simulink model "case1"  (R2024b)
settings: Solver=FixedStepAuto  StartTime=0  StopTime=1  FixedStep=1e-7  RelTol=1e-3
values from neighbouring files (symbols this model uses):
  SG_D_1_D = 0.01056    [IEEE9_case_parameters.m]    (also in case1_parameters.m; case2_parameters.m; case3_parameters.m; case4_parameters.m)
  SG_D_1_EnableSaturation = 0    [IEEE9_case_parameters.m]    (also in case1_parameters.m; case2_parameters.m; case3_parameters.m; case4_parameters.m)
  SG_D_1_f0 = 60    [IEEE9_case_parameters.m]    (also in case1_parameters.m; case2_parameters.m; case3_parameters.m; case4_parameters.m)
  SG_D_1_H = 7.5    [IEEE9_case_parameters.m]    (also in case1_parameters.m; case2_parameters.m; case3_parameters.m; case4_parameters.m)
  SG_D_1_K_A = 20    [IEEE9_case_parameters.m]    (also in case1_parameters.m; case2_parameters.m; case3_parameters.m; case4_parameters.m)
  SG_D_1_K_E = 1.000000e+1    (= 10)    [IEEE9_case_parameters.m]    (also in case1_parameters.m; case2_parameters.m; case3_parameters.m; case4_parameters.m)
  SG_D_1_K_F = 2.363    [IEEE9_case_parameters.m]    (also in case1_parameters.m; case2_parameters.m; case3_parameters.m; case4_parameters.m)
  SG_D_1_K_s = 0.5    [IEEE9_case_parameters.m]    (also in case1_parameters.m = 5; case2_parameters.m = 5; case3_parameters.m = 5; case4_parameters.m = 5)
  SG_D_1_R_a = 0.001088    [IEEE9_case_parameters.m]    (also in case1_parameters.m; case2_parameters.m; case3_parameters.m; case4_parameters.m)
  SG_D_1_S_A = 1    [IEEE9_case_parameters.m]    (also in case1_parameters.m; case2_parameters.m; case3_parameters.m; case4_parameters.m)
  SG_D_1_S_B = 0.103    [IEEE9_case_parameters.m]    (also in case1_parameters.m; case2_parameters.m; case3_parameters.m; case4_parameters.m)
  SG_D_1_S_N = 10.659857    [IEEE9_case_parameters.m]    (also in case1_parameters.m; case2_parameters.m; case3_parameters.m; case4_parameters.m)
  SG_D_1_SpeedPara = 200    [IEEE9_case_parameters.m]    (also in case1_parameters.m; case2_parameters.m; case3_parameters.m; case4_parameters.m)
  SG_D_1_T_0 = 0.720173    [IEEE9_case_parameters.m]    (also in case1_parameters.m = 0.755522; case2_parameters.m = 0.808931; case3_parameters.m = 0.869402; case4_parameters.m = 0.729316)
  SG_D_1_T_1 = 0.3    [IEEE9_case_parameters.m]    (also in case1_parameters.m; case2_parameters.m; case3_parameters.m; case4_parameters.m)
  SG_D_1_T_2 = 0.05    [IEEE9_case_parameters.m]    (also in case1_parameters.m; case2_parameters.m; case3_parameters.m; case4_parameters.m)
  SG_D_1_T_3 = 0.02    [IEEE9_case_parameters.m]    (also in case1_parameters.m; case2_parameters.m; case3_parameters.m; case4_parameters.m)
  SG_D_1_T_4 = 0.005    [IEEE9_case_parameters.m]    (also in case1_parameters.m; case2_parameters.m; case3_parameters.m; case4_parameters.m)
  SG_D_1_T_A = 0.02    [IEEE9_case_parameters.m]    (also in case1_parameters.m; case2_parameters.m; case3_parameters.m; case4_parameters.m)
  SG_D_1_T_dd = 8.000000e+0    (= 8)    [IEEE9_case_parameters.m]    (also in case1_parameters.m; case2_parameters.m; case3_parameters.m; case4_parameters.m)
  SG_D_1_T_ddd = 0.04    [IEEE9_case_parameters.m]    (also in case1_parameters.m; case2_parameters.m; case3_parameters.m; case4_parameters.m)
  SG_D_1_T_E = 0.314    [IEEE9_case_parameters.m]    (also in case1_parameters.m; case2_parameters.m; case3_parameters.m; case4_parameters.m)
  SG_D_1_T_F = 0.35    [IEEE9_case_parameters.m]    (also in case1_parameters.m; case2_parameters.m; case3_parameters.m; case4_parameters.m)
  SG_D_1_T_qd = 0.8    [IEEE9_case_parameters.m]    (also in case1_parameters.m; case2_parameters.m; case3_parameters.m; case4_parameters.m)
  SG_D_1_T_qdd = 0.02    [IEEE9_case_parameters.m]    (also in case1_parameters.m; case2_parameters.m; case3_parameters.m; case4_parameters.m)
  SG_D_1_T_speed = 0.1    [IEEE9_case_parameters.m]    (also in case1_parameters.m = 200; case2_parameters.m = 200; case3_parameters.m = 200; case4_parameters.m = 200)
  SG_D_1_T_w = 0.5    [IEEE9_case_parameters.m]    (also in case1_parameters.m; case2_parameters.m; case3_parameters.m; case4_parameters.m)
  SG_D_1_V_ref = 1.990276    [IEEE9_case_parameters.m]    (also in case1_parameters.m = 2.042296; case2_parameters.m = 2.051388; case3_parameters.m = 2.089584; case4_parameters.m = 2.01845)
  SG_D_1_w_ref = 376.991118    [IEEE9_case_parameters.m]    (also in case1_parameters.m; case2_parameters.m; case3_parameters.m; case4_parameters.m)
  SG_D_1_wb = 6.000000e+1    (= 60)    [IEEE9_case_parameters.m]    (also in case1_parameters.m; case2_parameters.m; case3_parameters.m; case4_parameters.m)
  SG_D_1_x_d = 1.9    [IEEE9_case_parameters.m]    (also in case1_parameters.m; case2_parameters.m; case3_parameters.m; case4_parameters.m)
  SG_D_1_x_dd = 0.302    [IEEE9_case_parameters.m]    (also in case1_parameters.m; case2_parameters.m; case3_parameters.m; case4_parameters.m)
  SG_D_1_x_ddd = 0.204    [IEEE9_case_parameters.m]    (also in case1_parameters.m; case2_parameters.m; case3_parameters.m; case4_parameters.m)
  SG_D_1_x_l = 0.05    [IEEE9_case_parameters.m]    (also in case1_parameters.m; case2_parameters.m; case3_parameters.m; case4_parameters.m)
  SG_D_1_x_q = 1.3    [IEEE9_case_parameters.m]    (also in case1_parameters.m; case2_parameters.m; case3_parameters.m; case4_parameters.m)
  SG_D_1_x_qd = 0.5    [IEEE9_case_parameters.m]    (also in case1_parameters.m; case2_parameters.m; case3_parameters.m; case4_parameters.m)
  SG_D_1_x_qdd = 0.3    [IEEE9_case_parameters.m]    (also in case1_parameters.m; case2_parameters.m; case3_parameters.m; case4_parameters.m)
  SG_D_2_D = 0.02    [IEEE9_case_parameters.m]    (also in case1_parameters.m; case2_parameters.m; case3_parameters.m; case4_parameters.m)
  SG_D_2_EnableSaturation = 0    [IEEE9_case_parameters.m]    (also in case1_parameters.m; case2_parameters.m; case3_parameters.m; case4_parameters.m)
  SG_D_2_f0 = 60    [IEEE9_case_parameters.m]    (also in case1_parameters.m; case2_parameters.m; case3_parameters.m; case4_parameters.m)
  SG_D_2_H = 8.000000e+0    (= 8)    [IEEE9_case_parameters.m]    (also in case1_parameters.m; case2_parameters.m; case3_parameters.m; case4_parameters.m)
  SG_D_2_K_A = 20    [IEEE9_case_parameters.m]    (also in case1_parameters.m; case2_parameters.m; case3_parameters.m; case4_parameters.m)
  SG_D_2_K_E = 1.000000e+1    (= 10)    [IEEE9_case_parameters.m]    (also in case1_parameters.m; case2_parameters.m; case3_parameters.m; case4_parameters.m)
  SG_D_2_K_F = 2.363    [IEEE9_case_parameters.m]    (also in case1_parameters.m; case2_parameters.m; case3_parameters.m; case4_parameters.m)
  SG_D_2_K_s = 0.5    [IEEE9_case_parameters.m]    (also in case1_parameters.m = 4; case2_parameters.m = 4; case3_parameters.m = 4; case4_parameters.m = 4)
  SG_D_2_R_a = 0.001088    [IEEE9_case_parameters.m]    (also in case1_parameters.m; case2_parameters.m; case3_parameters.m; case4_parameters.m)
  SG_D_2_S_A = 1    [IEEE9_case_parameters.m]    (also in case1_parameters.m; case2_parameters.m; case3_parameters.m; case4_parameters.m)
  SG_D_2_S_B = 0.103    [IEEE9_case_parameters.m]    (also in case1_parameters.m; case2_parameters.m; case3_parameters.m; case4_parameters.m)
  SG_D_2_S_N = 10.659857    [IEEE9_case_parameters.m]    (also in case1_parameters.m; case2_parameters.m; case3_parameters.m; case4_parameters.m)
  SG_D_2_SpeedPara = 200    [IEEE9_case_parameters.m]    (also in case1_parameters.m; case2_parameters.m; case3_parameters.m; case4_parameters.m)
  SG_D_2_T_0 = 1.632913    [IEEE9_case_parameters.m]    (also in case1_parameters.m = 1.632925; case2_parameters.m = 1.632915; case3_parameters.m = 1.632914; case4_parameters.m = 1.632927)
  SG_D_2_T_1 = 0.2    [IEEE9_case_parameters.m]    (also in case1_parameters.m; case2_parameters.m; case3_parameters.m; case4_parameters.m)
  SG_D_2_T_2 = 0.05    [IEEE9_case_parameters.m]    (also in case1_parameters.m; case2_parameters.m; case3_parameters.m; case4_parameters.m)
  SG_D_2_T_3 = 0.02    [IEEE9_case_parameters.m]    (also in case1_parameters.m; case2_parameters.m; case3_parameters.m; case4_parameters.m)
  SG_D_2_T_4 = 0.005    [IEEE9_case_parameters.m]    (also in case1_parameters.m; case2_parameters.m; case3_parameters.m; case4_parameters.m)
  SG_D_2_T_A = 0.02    [IEEE9_case_parameters.m]    (also in case1_parameters.m; case2_parameters.m; case3_parameters.m; case4_parameters.m)
  SG_D_2_T_dd = 7.9    [IEEE9_case_parameters.m]    (also in case1_parameters.m; case2_parameters.m; case3_parameters.m; case4_parameters.m)
  SG_D_2_T_ddd = 0.04    [IEEE9_case_parameters.m]    (also in case1_parameters.m; case2_parameters.m; case3_parameters.m; case4_parameters.m)
  SG_D_2_T_E = 0.314    [IEEE9_case_parameters.m]    (also in case1_parameters.m; case2_parameters.m; case3_parameters.m; case4_parameters.m)
  SG_D_2_T_F = 0.35    [IEEE9_case_parameters.m]    (also in case1_parameters.m; case2_parameters.m; case3_parameters.m; case4_parameters.m)
  SG_D_2_T_qd = 0.8    [IEEE9_case_parameters.m]    (also in case1_parameters.m; case2_parameters.m; case3_parameters.m; case4_parameters.m)
  SG_D_2_T_qdd = 0.015    [IEEE9_case_parameters.m]    (also in case1_parameters.m; case2_parameters.m; case3_parameters.m; case4_parameters.m)
  SG_D_2_T_speed = 0.1    [IEEE9_case_parameters.m]    (also in case1_parameters.m = 150; case2_parameters.m = 150; case3_parameters.m = 150; case4_parameters.m = 150)
  SG_D_2_T_w = 0.35    [IEEE9_case_parameters.m]    (also in case1_parameters.m; case2_parameters.m; case3_parameters.m; case4_parameters.m)
  SG_D_2_V_ref = 2.58547    [IEEE9_case_parameters.m]    (also in case1_parameters.m = 2.597896; case2_parameters.m = 2.587136; case3_parameters.m = 2.586042; case4_parameters.m = 2.599679)
  SG_D_2_w_ref = 376.991118    [IEEE9_case_parameters.m]    (also in case1_parameters.m; case2_parameters.m; case3_parameters.m; case4_parameters.m)
  SG_D_2_wb = 6.000000e+1    (= 60)    [IEEE9_case_parameters.m]    (also in case1_parameters.m; case2_parameters.m; case3_parameters.m; case4_parameters.m)
  SG_D_2_x_d = 1.8    [IEEE9_case_parameters.m]    (also in case1_parameters.m; case2_parameters.m; case3_parameters.m; case4_parameters.m)
  SG_D_2_x_dd = 0.302    [IEEE9_case_parameters.m]    (also in case1_parameters.m; case2_parameters.m; case3_parameters.m; case4_parameters.m)
  SG_D_2_x_ddd = 0.204    [IEEE9_case_parameters.m]    (also in case1_parameters.m; case2_parameters.m; case3_parameters.m; case4_parameters.m)
  SG_D_2_x_l = 0.05    [IEEE9_case_parameters.m]    (also in case1_parameters.m; case2_parameters.m; case3_parameters.m; case4_parameters.m)
  SG_D_2_x_q = 1.25    [IEEE9_case_parameters.m]    (also in case1_parameters.m; case2_parameters.m; case3_parameters.m; case4_parameters.m)
  SG_D_2_x_qd = 0.5    [IEEE9_case_parameters.m]    (also in case1_parameters.m; case2_parameters.m; case3_parameters.m; case4_parameters.m)
  SG_D_2_x_qdd = 0.3    [IEEE9_case_parameters.m]    (also in case1_parameters.m; case2_parameters.m; case3_parameters.m; case4_parameters.m)
  SG_D_3_D = 0.02    [IEEE9_case_parameters.m]    (also in case1_parameters.m; case2_parameters.m; case3_parameters.m; case4_parameters.m)
  SG_D_3_EnableSaturation = 0    [IEEE9_case_parameters.m]    (also in case1_parameters.m; case2_parameters.m; case3_parameters.m; case4_parameters.m)
  SG_D_3_f0 = 60    [IEEE9_case_parameters.m]    (also in case1_parameters.m; case2_parameters.m; case3_parameters.m; case4_parameters.m)
  SG_D_3_H = 7.7    [IEEE9_case_parameters.m]    (also in case1_parameters.m; case2_parameters.m; case3_parameters.m; case4_parameters.m)
  SG_D_3_K_A = 20    [IEEE9_case_parameters.m]    (also in case1_parameters.m; case2_parameters.m; case3_parameters.m; case4_parameters.m)
  SG_D_3_K_E = 1.000000e+1    (= 10)    [IEEE9_case_parameters.m]    (also in case1_parameters.m; case2_parameters.m; case3_parameters.m; case4_parameters.m)
  SG_D_3_K_F = 2.363    [IEEE9_case_parameters.m]    (also in case1_parameters.m; case2_parameters.m; case3_parameters.m; case4_parameters.m)
  SG_D_3_K_s = 0.2    [IEEE9_case_parameters.m]    (also in case1_parameters.m = 2; case2_parameters.m = 2; case3_parameters.m = 2; case4_parameters.m = 2)
  SG_D_3_R_a = 0.001088    [IEEE9_case_parameters.m]    (also in case1_parameters.m; case2_parameters.m; case3_parameters.m; case4_parameters.m)
  SG_D_3_S_A = 1    [IEEE9_case_parameters.m]    (also in case1_parameters.m; case2_parameters.m; case3_parameters.m; case4_parameters.m)
  SG_D_3_S_B = 0.103    [IEEE9_case_parameters.m]    (also in case1_parameters.m; case2_parameters.m; case3_parameters.m; case4_parameters.m)
  SG_D_3_S_N = 10.659857    [IEEE9_case_parameters.m]    (also in case1_parameters.m; case2_parameters.m; case3_parameters.m; case4_parameters.m)
  SG_D_3_SpeedPara = 200    [IEEE9_case_parameters.m]    (also in case1_parameters.m; case2_parameters.m; case3_parameters.m; case4_parameters.m)
  SG_D_3_T_0 = 0.850788    [IEEE9_case_parameters.m]    (also in case1_parameters.m = 0.850786; case2_parameters.m = 0.850787; case3_parameters.m; case4_parameters.m = 0.850786)
  SG_D_3_T_1 = 0.2    [IEEE9_case_parameters.m]    (also in case1_parameters.m; case2_parameters.m; case3_parameters.m; case4_parameters.m)
  SG_D_3_T_2 = 0.05    [IEEE9_case_parameters.m]    (also in case1_parameters.m; case2_parameters.m; case3_parameters.m; case4_parameters.m)
  SG_D_3_T_3 = 0.02    [IEEE9_case_parameters.m]    (also in case1_parameters.m; case2_parameters.m; case3_parameters.m; case4_parameters.m)
  SG_D_3_T_4 = 0.005    [IEEE9_case_parameters.m]    (also in case1_parameters.m; case2_parameters.m; case3_parameters.m; case4_parameters.m)
  SG_D_3_T_A = 0.02    [IEEE9_case_parameters.m]    (also in case1_parameters.m; case2_parameters.m; case3_parameters.m; case4_parameters.m)
  SG_D_3_T_dd = 8.1    [IEEE9_case_parameters.m]    (also in case1_parameters.m; case2_parameters.m; case3_parameters.m; case4_parameters.m)
  SG_D_3_T_ddd = 0.04    [IEEE9_case_parameters.m]    (also in case1_parameters.m; case2_parameters.m; case3_parameters.m; case4_parameters.m)
  SG_D_3_T_E = 0.314    [IEEE9_case_parameters.m]    (also in case1_parameters.m; case2_parameters.m; case3_parameters.m; case4_parameters.m)
  SG_D_3_T_F = 0.35    [IEEE9_case_parameters.m]    (also in case1_parameters.m; case2_parameters.m; case3_parameters.m; case4_parameters.m)
  SG_D_3_T_qd = 0.8    [IEEE9_case_parameters.m]    (also in case1_parameters.m; case2_parameters.m; case3_parameters.m; case4_parameters.m)
  SG_D_3_T_qdd = 0.015    [IEEE9_case_parameters.m]    (also in case1_parameters.m; case2_parameters.m; case3_parameters.m; case4_parameters.m)
  SG_D_3_T_speed = 0.1    [IEEE9_case_parameters.m]    (also in case1_parameters.m = 180; case2_parameters.m = 180; case3_parameters.m = 180; case4_parameters.m = 180)
  SG_D_3_T_w = 0.4    [IEEE9_case_parameters.m]    (also in case1_parameters.m; case2_parameters.m; case3_parameters.m; case4_parameters.m)
  SG_D_3_V_ref = 1.892727    [IEEE9_case_parameters.m]    (also in case1_parameters.m = 1.906439; case2_parameters.m = 1.895535; case3_parameters.m = 1.892105; case4_parameters.m = 1.906598)
  SG_D_3_w_ref = 376.991118    [IEEE9_case_parameters.m]    (also in case1_parameters.m; case2_parameters.m; case3_parameters.m; case4_parameters.m)
  SG_D_3_wb = 6.000000e+1    (= 60)    [IEEE9_case_parameters.m]    (also in case1_parameters.m; case2_parameters.m; case3_parameters.m; case4_parameters.m)
  SG_D_3_x_d = 1.85    [IEEE9_case_parameters.m]    (also in case1_parameters.m; case2_parameters.m; case3_parameters.m; case4_parameters.m)
  SG_D_3_x_dd = 0.302    [IEEE9_case_parameters.m]    (also in case1_parameters.m; case2_parameters.m; case3_parameters.m; case4_parameters.m)
  SG_D_3_x_ddd = 0.204    [IEEE9_case_parameters.m]    (also in case1_parameters.m; case2_parameters.m; case3_parameters.m; case4_parameters.m)
  SG_D_3_x_l = 0.05    [IEEE9_case_parameters.m]    (also in case1_parameters.m; case2_parameters.m; case3_parameters.m; case4_parameters.m)
  SG_D_3_x_q = 1.2    [IEEE9_case_parameters.m]    (also in case1_parameters.m; case2_parameters.m; case3_parameters.m; case4_parameters.m)
  SG_D_3_x_qd = 0.5    [IEEE9_case_parameters.m]    (also in case1_parameters.m; case2_parameters.m; case3_parameters.m; case4_parameters.m)
  SG_D_3_x_qdd = 0.3    [IEEE9_case_parameters.m]    (also in case1_parameters.m; case2_parameters.m; case3_parameters.m; case4_parameters.m)
(part 4 of 12)

== system case1/AC_1/d_vq_bus_7_block ==
  note: d_vq_bus_7 in case1
      | $2106.09563369148\,\mathrm{iq}_{\mathrm{bus},7}-376.991118430775\,\mathrm{vd}_{\mathrm{bus},7}$
      | Automatically generated on 2025-10-31 18:50:31 .
  Alge_iq_bus_7_85db4 : Inport
  State_vd_bus_7_89a44 : Inport  Port=2
  Constant_2106.09563369148_3c2f9 : Constant  Value=2106.09563369148
  Constant_376.991118430775_5ea0f : Constant  Value=376.991118430775
  Product_081df : Product
  Product_b1f89 : Product
  Subtract_831b9 : Sum  Inputs=+-
  Blockout_d_vq_bus_7_1fb71 : Outport
  wires:
  Constant_2106.09563369148_3c2f9/1 -> Product_b1f89/1
  Product_081df/1 -> Subtract_831b9/2
  Alge_iq_bus_7_85db4/1 -> Product_b1f89/2
  Constant_376.991118430775_5ea0f/1 -> Product_081df/1
  Subtract_831b9/1 -> Blockout_d_vq_bus_7_1fb71/1
  State_vd_bus_7_89a44/1 -> Product_081df/2
  Product_b1f89/1 -> Subtract_831b9/1

== system case1/AC_1/d_vq_bus_8_block ==
  note: d_vq_bus_8 in case1
      | $1657.10381727813\,\mathrm{iq}_{\mathrm{bus},8}-376.991118430775\,\mathrm{vd}_{\mathrm{bus},8}$
      | Automatically generated on 2025-10-31 18:50:33 .
  Alge_iq_bus_8_dc6f7 : Inport
  State_vd_bus_8_2280e : Inport  Port=2
  Constant_1657.10381727813_7ad0e : Constant  Value=1657.10381727813
  Constant_376.991118430775_f83d7 : Constant  Value=376.991118430775
  Product_3832f : Product
  Product_65f65 : Product
  Subtract_b2c39 : Sum  Inputs=+-
  Blockout_d_vq_bus_8_79652 : Outport
  wires:
  Constant_1657.10381727813_7ad0e/1 -> Product_65f65/1
  Constant_376.991118430775_f83d7/1 -> Product_3832f/1
  Alge_iq_bus_8_dc6f7/1 -> Product_65f65/2
  State_vd_bus_8_2280e/1 -> Product_3832f/2
  Product_65f65/1 -> Subtract_b2c39/1
  Product_3832f/1 -> Subtract_b2c39/2
  Subtract_b2c39/1 -> Blockout_d_vq_bus_8_79652/1

== system case1/AC_1/d_vq_bus_9_block ==
  note: d_vq_bus_9 in case1
      | $1564.27849971276\,\mathrm{iq}_{\mathrm{bus},9}-376.991118430775\,\mathrm{vd}_{\mathrm{bus},9}$
      | Automatically generated on 2025-10-31 18:50:35 .
  Alge_iq_bus_9_ce7a0 : Inport
  State_vd_bus_9_7cb95 : Inport  Port=2
  Constant_1564.27849971276_fd290 : Constant  Value=1564.27849971276
  Constant_376.991118430775_417d9 : Constant  Value=376.991118430775
  Product_93a7f : Product
  Product_c24f3 : Product
  Subtract_d6f5e : Sum  Inputs=+-
  Blockout_d_vq_bus_9_cbc85 : Outport
  wires:
  Constant_1564.27849971276_fd290/1 -> Product_93a7f/1
  Constant_376.991118430775_417d9/1 -> Product_c24f3/1
  Alge_iq_bus_9_ce7a0/1 -> Product_93a7f/2
  State_vd_bus_9_7cb95/1 -> Product_c24f3/2
  Product_93a7f/1 -> Subtract_d6f5e/1
  Product_c24f3/1 -> Subtract_d6f5e/2
  Subtract_d6f5e/1 -> Blockout_d_vq_bus_9_cbc85/1

== system case1/AC_1/id_bus_1_block ==
  note: id_bus_1 in case1
      | $\mathrm{id}_{\mathrm{SG},D,1}-\mathrm{id}_{\mathrm{line},1,4}$
      | Automatically generated on 2025-10-31 18:51:04 .
  Input_id_SG_D_1_23990 : Inport
  State_id_line_1_4_dac35 : Inport  Port=2
  Subtract_53f6c : Sum  Inputs=+-
  Blockout_id_bus_1_33f85 : Outport
  wires:
  Input_id_SG_D_1_23990/1 -> Subtract_53f6c/1
  State_id_line_1_4_dac35/1 -> Subtract_53f6c/2
  Subtract_53f6c/1 -> Blockout_id_bus_1_33f85/1

== system case1/AC_1/id_bus_2_block ==
  note: id_bus_2 in case1
      | $\mathrm{id}_{\mathrm{SG},D,2}+\mathrm{id}_{\mathrm{line},8,2}$
      | Automatically generated on 2025-10-31 18:51:07 .
  Input_id_SG_D_2_52bf0 : Inport
  State_id_line_8_2_e06f3 : Inport  Port=2
  Add_2cb8d : Sum
  Blockout_id_bus_2_bdcc8 : Outport
  wires:
  Input_id_SG_D_2_52bf0/1 -> Add_2cb8d/1
  State_id_line_8_2_e06f3/1 -> Add_2cb8d/2
  Add_2cb8d/1 -> Blockout_id_bus_2_bdcc8/1

== system case1/AC_1/id_bus_3_block ==
  note: id_bus_3 in case1
      | $\mathrm{id}_{\mathrm{SG},D,3}-\mathrm{id}_{\mathrm{line},3,6}$
      | Automatically generated on 2025-10-31 18:51:09 .
  Input_id_SG_D_3_c7560 : Inport
  State_id_line_3_6_bccaf : Inport  Port=2
  Subtract_0a38c : Sum  Inputs=+-
  Blockout_id_bus_3_3aea8 : Outport
  wires:
  Input_id_SG_D_3_c7560/1 -> Subtract_0a38c/1
  State_id_line_3_6_bccaf/1 -> Subtract_0a38c/2
  Subtract_0a38c/1 -> Blockout_id_bus_3_3aea8/1

== system case1/AC_1/id_bus_4_block ==
  note: id_bus_4 in case1
      | $\mathrm{id}_{\mathrm{line},1,4}-\mathrm{id}_{\mathrm{line},4,5}+\mathrm{id}_{\mathrm{line},9,4}$
      | Automatically generated on 2025-10-31 18:51:10 .
  State_id_line_1_4_58bbd : Inport
  State_id_line_4_5_ac403 : Inport  Port=2
  State_id_line_9_4_ed76d : Inport  Port=3
  Add_53c6e : Sum
  Subtract_51822 : Sum  Inputs=+-
  Blockout_id_bus_4_e4a8c : Outport
  wires:
  State_id_line_9_4_ed76d/1 -> Add_53c6e/2
  State_id_line_1_4_58bbd/1 -> Subtract_51822/1
  State_id_line_4_5_ac403/1 -> Subtract_51822/2
  Subtract_51822/1 -> Add_53c6e/1
  Add_53c6e/1 -> Blockout_id_bus_4_e4a8c/1

== system case1/AC_1/id_bus_5_block ==
  note: id_bus_5 in case1
      | $\mathrm{id}_{\mathrm{line},4,5}-\mathrm{id}_{\mathrm{load},5}-\mathrm{id}_{\mathrm{line},5,6}$
      | Automatically generated on 2025-10-31 18:51:12 .
  State_id_load_5_329c5 : Inport
  State_id_line_4_5_8dac8 : Inport  Port=2
  State_id_line_5_6_8622f : Inport  Port=3
  Add_9d10b : Sum
  Constant_-1_d2515 : Constant  Value=-1
  Product_b5f46 : Product
  Subtract_cf589 : Sum  Inputs=+-
  Blockout_id_bus_5_517a7 : Outport
  wires:
  Subtract_cf589/1 -> Blockout_id_bus_5_517a7/1
  State_id_line_4_5_8dac8/1 -> Add_9d10b/2
  Constant_-1_d2515/1 -> Product_b5f46/1
  Add_9d10b/1 -> Subtract_cf589/1
  State_id_load_5_329c5/1 -> Product_b5f46/2
  Product_b5f46/1 -> Add_9d10b/1
  State_id_line_5_6_8622f/1 -> Subtract_cf589/2

== system case1/AC_1/id_bus_6_block ==
  note: id_bus_6 in case1
      | $\mathrm{id}_{\mathrm{line},3,6}+\mathrm{id}_{\mathrm{line},5,6}-\mathrm{id}_{\mathrm{line},6,7}$
      | Automatically generated on 2025-10-31 18:51:14 .
  State_id_line_3_6_274c1 : Inport
  State_id_line_5_6_a25b6 : Inport  Port=2
  State_id_line_6_7_bc3d2 : Inport  Port=3
  Add_da054 : Sum
  Subtract_7521e : Sum  Inputs=+-
  Blockout_id_bus_6_229a8 : Outport
  wires:
  State_id_line_6_7_bc3d2/1 -> Subtract_7521e/2
  State_id_line_3_6_274c1/1 -> Add_da054/1
  State_id_line_5_6_a25b6/1 -> Add_da054/2
  Add_da054/1 -> Subtract_7521e/1
  Subtract_7521e/1 -> Blockout_id_bus_6_229a8/1

== system case1/AC_1/id_bus_7_block ==
  note: id_bus_7 in case1
      | $\mathrm{id}_{\mathrm{line},6,7}-\mathrm{id}_{\mathrm{load},7}-\mathrm{id}_{\mathrm{line},7,8}$
      | Automatically generated on 2025-10-31 18:51:15 .
  State_id_load_7_eaed7 : Inport
  State_id_line_6_7_ab1bc : Inport  Port=2
  State_id_line_7_8_5b752 : Inport  Port=3
  Add_2bb96 : Sum
  Constant_-1_57f2b : Constant  Value=-1
  Product_e05be : Product
  Subtract_eedde : Sum  Inputs=+-
  Blockout_id_bus_7_b6ff1 : Outport
  wires:
  Subtract_eedde/1 -> Blockout_id_bus_7_b6ff1/1
  State_id_line_6_7_ab1bc/1 -> Add_2bb96/2
  Constant_-1_57f2b/1 -> Product_e05be/1
  Add_2bb96/1 -> Subtract_eedde/1
  State_id_load_7_eaed7/1 -> Product_e05be/2
  Product_e05be/1 -> Add_2bb96/1
  State_id_line_7_8_5b752/1 -> Subtract_eedde/2

== system case1/AC_1/id_bus_8_block ==
  note: id_bus_8 in case1
      | $\mathrm{id}_{\mathrm{line},7,8}-\mathrm{id}_{\mathrm{line},8,2}-\mathrm{id}_{\mathrm{line},8,9}$
      | Automatically generated on 2025-10-31 18:51:17 .
  State_id_line_7_8_3ae3c : Inport
  State_id_line_8_2_8ae43 : Inport  Port=2
  State_id_line_8_9_9335c : Inport  Port=3
  Subtract_4d2d2 : Sum  Inputs=+-
  Subtract_bca9f : Sum  Inputs=+-
  Blockout_id_bus_8_9838c : Outport
  wires:
  State_id_line_8_9_9335c/1 -> Subtract_4d2d2/2
  State_id_line_7_8_3ae3c/1 -> Subtract_bca9f/1
  State_id_line_8_2_8ae43/1 -> Subtract_bca9f/2
  Subtract_bca9f/1 -> Subtract_4d2d2/1
  Subtract_4d2d2/1 -> Blockout_id_bus_8_9838c/1

== system case1/AC_1/id_bus_9_block ==
  note: id_bus_9 in case1
      | $\mathrm{id}_{\mathrm{line},8,9}-\mathrm{id}_{\mathrm{load},9}-\mathrm{id}_{\mathrm{line},9,4}$
      | Automatically generated on 2025-10-31 18:51:19 .
  State_id_load_9_d5952 : Inport
  State_id_line_8_9_b8e8c : Inport  Port=2
  State_id_line_9_4_85e6f : Inport  Port=3
  Add_c7479 : Sum
  Constant_-1_c8019 : Constant  Value=-1
  Product_9d9a4 : Product
  Subtract_80fc7 : Sum  Inputs=+-
  Blockout_id_bus_9_d8517 : Outport
  wires:
  Subtract_80fc7/1 -> Blockout_id_bus_9_d8517/1
  State_id_line_8_9_b8e8c/1 -> Add_c7479/2
  Constant_-1_c8019/1 -> Product_9d9a4/1
  Add_c7479/1 -> Subtract_80fc7/1
  State_id_load_9_d5952/1 -> Product_9d9a4/2
  Product_9d9a4/1 -> Add_c7479/1
  State_id_line_9_4_85e6f/1 -> Subtract_80fc7/2

== system case1/AC_1/iq_bus_1_block ==
  note: iq_bus_1 in case1
      | $\mathrm{iq}_{\mathrm{SG},D,1}-\mathrm{iq}_{\mathrm{line},1,4}$
      | Automatically generated on 2025-10-31 18:51:05 .
  Input_iq_SG_D_1_6fe57 : Inport
  State_iq_line_1_4_19711 : Inport  Port=2
  Subtract_11345 : Sum  Inputs=+-
  Blockout_iq_bus_1_a9d09 : Outport
  wires:
  Input_iq_SG_D_1_6fe57/1 -> Subtract_11345/1
  State_iq_line_1_4_19711/1 -> Subtract_11345/2
  Subtract_11345/1 -> Blockout_iq_bus_1_a9d09/1

== system case1/AC_1/iq_bus_2_block ==
  note: iq_bus_2 in case1
      | $\mathrm{iq}_{\mathrm{SG},D,2}+\mathrm{iq}_{\mathrm{line},8,2}$
      | Automatically generated on 2025-10-31 18:51:07 .
  Input_iq_SG_D_2_5d5eb : Inport
  State_iq_line_8_2_b9f43 : Inport  Port=2
  Add_3b501 : Sum
  Blockout_iq_bus_2_a400f : Outport
  wires:
  Input_iq_SG_D_2_5d5eb/1 -> Add_3b501/1
  State_iq_line_8_2_b9f43/1 -> Add_3b501/2
  Add_3b501/1 -> Blockout_iq_bus_2_a400f/1

== system case1/AC_1/iq_bus_3_block ==
  note: iq_bus_3 in case1
      | $\mathrm{iq}_{\mathrm{SG},D,3}-\mathrm{iq}_{\mathrm{line},3,6}$
      | Automatically generated on 2025-10-31 18:51:10 .
  Input_iq_SG_D_3_98297 : Inport
  State_iq_line_3_6_41bc5 : Inport  Port=2
  Subtract_be933 : Sum  Inputs=+-
  Blockout_iq_bus_3_1800f : Outport
  wires:
  Input_iq_SG_D_3_98297/1 -> Subtract_be933/1
  State_iq_line_3_6_41bc5/1 -> Subtract_be933/2
  Subtract_be933/1 -> Blockout_iq_bus_3_1800f/1

== system case1/AC_1/iq_bus_4_block ==
  note: iq_bus_4 in case1
      | $\mathrm{iq}_{\mathrm{line},1,4}-\mathrm{iq}_{\mathrm{line},4,5}+\mathrm{iq}_{\mathrm{line},9,4}$
      | Automatically generated on 2025-10-31 18:51:11 .
  State_iq_line_1_4_208ce : Inport
  State_iq_line_4_5_c03c7 : Inport  Port=2
  State_iq_line_9_4_b5c11 : Inport  Port=3
  Add_a8f90 : Sum
  Subtract_3b5cd : Sum  Inputs=+-
  Blockout_iq_bus_4_f7785 : Outport
  wires:
  State_iq_line_1_4_208ce/1 -> Subtract_3b5cd/1
  State_iq_line_4_5_c03c7/1 -> Subtract_3b5cd/2
  Subtract_3b5cd/1 -> Add_a8f90/1
  State_iq_line_9_4_b5c11/1 -> Add_a8f90/2
  Add_a8f90/1 -> Blockout_iq_bus_4_f7785/1

== system case1/AC_1/iq_bus_5_block ==
  note: iq_bus_5 in case1
      | $\mathrm{iq}_{\mathrm{line},4,5}-\mathrm{iq}_{\mathrm{load},5}-\mathrm{iq}_{\mathrm{line},5,6}$
      | Automatically generated on 2025-10-31 18:51:13 .
  State_iq_load_5_fd86e : Inport
  State_iq_line_4_5_29371 : Inport  Port=2
  State_iq_line_5_6_b096e : Inport  Port=3
  Add_2dccb : Sum
  Constant_-1_46fd0 : Constant  Value=-1
  Product_4eb8e : Product
  Subtract_d2eac : Sum  Inputs=+-
  Blockout_iq_bus_5_6e2a7 : Outport
  wires:
  Subtract_d2eac/1 -> Blockout_iq_bus_5_6e2a7/1
  State_iq_line_4_5_29371/1 -> Add_2dccb/2
  Constant_-1_46fd0/1 -> Product_4eb8e/1
  State_iq_load_5_fd86e/1 -> Product_4eb8e/2
  Product_4eb8e/1 -> Add_2dccb/1
  Add_2dccb/1 -> Subtract_d2eac/1
  State_iq_line_5_6_b096e/1 -> Subtract_d2eac/2

== system case1/AC_1/iq_bus_6_block ==
  note: iq_bus_6 in case1
      | $\mathrm{iq}_{\mathrm{line},3,6}+\mathrm{iq}_{\mathrm{line},5,6}-\mathrm{iq}_{\mathrm{line},6,7}$
      | Automatically generated on 2025-10-31 18:51:14 .
  State_iq_line_3_6_b594c : Inport
  State_iq_line_5_6_ff608 : Inport  Port=2
  State_iq_line_6_7_100bb : Inport  Port=3
  Add_ba085 : Sum
  Subtract_747a3 : Sum  Inputs=+-
  Blockout_iq_bus_6_b8b39 : Outport
  wires:
  State_iq_line_3_6_b594c/1 -> Add_ba085/1
  State_iq_line_5_6_ff608/1 -> Add_ba085/2
  Add_ba085/1 -> Subtract_747a3/1
  State_iq_line_6_7_100bb/1 -> Subtract_747a3/2
  Subtract_747a3/1 -> Blockout_iq_bus_6_b8b39/1

== system case1/AC_1/iq_bus_7_block ==
  note: iq_bus_7 in case1
      | $\mathrm{iq}_{\mathrm{line},6,7}-\mathrm{iq}_{\mathrm{load},7}-\mathrm{iq}_{\mathrm{line},7,8}$
      | Automatically generated on 2025-10-31 18:51:16 .
  State_iq_load_7_b0e2f : Inport
  State_iq_line_6_7_6bc6f : Inport  Port=2
  State_iq_line_7_8_d005c : Inport  Port=3
  Add_5dd0b : Sum
  Constant_-1_bef7d : Constant  Value=-1
  Product_701d1 : Product
  Subtract_8275f : Sum  Inputs=+-
  Blockout_iq_bus_7_2e710 : Outport
  wires:
  Subtract_8275f/1 -> Blockout_iq_bus_7_2e710/1
  State_iq_line_6_7_6bc6f/1 -> Add_5dd0b/2
  Constant_-1_bef7d/1 -> Product_701d1/1
  State_iq_load_7_b0e2f/1 -> Product_701d1/2
  Product_701d1/1 -> Add_5dd0b/1
  Add_5dd0b/1 -> Subtract_8275f/1
  State_iq_line_7_8_d005c/1 -> Subtract_8275f/2

== system case1/AC_1/iq_bus_8_block ==
  note: iq_bus_8 in case1
      | $\mathrm{iq}_{\mathrm{line},7,8}-\mathrm{iq}_{\mathrm{line},8,2}-\mathrm{iq}_{\mathrm{line},8,9}$
      | Automatically generated on 2025-10-31 18:51:18 .
  State_iq_line_7_8_4bd2e : Inport
  State_iq_line_8_2_22f52 : Inport  Port=2
  State_iq_line_8_9_4f885 : Inport  Port=3
  Subtract_236a4 : Sum  Inputs=+-
  Subtract_8641d : Sum  Inputs=+-
  Blockout_iq_bus_8_1bc28 : Outport
  wires:
  State_iq_line_7_8_4bd2e/1 -> Subtract_8641d/1
  State_iq_line_8_2_22f52/1 -> Subtract_8641d/2
  Subtract_8641d/1 -> Subtract_236a4/1
  State_iq_line_8_9_4f885/1 -> Subtract_236a4/2
  Subtract_236a4/1 -> Blockout_iq_bus_8_1bc28/1

== system case1/AC_1/iq_bus_9_block ==
  note: iq_bus_9 in case1
      | $\mathrm{iq}_{\mathrm{line},8,9}-\mathrm{iq}_{\mathrm{load},9}-\mathrm{iq}_{\mathrm{line},9,4}$
      | Automatically generated on 2025-10-31 18:51:20 .
  State_iq_load_9_04094 : Inport
  State_iq_line_8_9_2cb5f : Inport  Port=2
  State_iq_line_9_4_7546b : Inport  Port=3
  Add_2e44f : Sum
  Constant_-1_168d4 : Constant  Value=-1
  Product_67ffe : Product
  Subtract_17b27 : Sum  Inputs=+-
  Blockout_iq_bus_9_07c34 : Outport
  wires:
  Subtract_17b27/1 -> Blockout_iq_bus_9_07c34/1
  State_iq_line_8_9_2cb5f/1 -> Add_2e44f/2
  Constant_-1_168d4/1 -> Product_67ffe/1
  State_iq_load_9_04094/1 -> Product_67ffe/2
  Product_67ffe/1 -> Add_2e44f/1
  Add_2e44f/1 -> Subtract_17b27/1
  State_iq_line_9_4_7546b/1 -> Subtract_17b27/2

== system case1/AC_1/vd_bus_1_out_block ==
  note: vd_bus_1_out in case1
      | $\mathrm{vd}_{\mathrm{bus},1}$
      | Automatically generated on 2025-10-31 18:51:03 .
  State_vd_bus_1_cf04b : Inport
  Blockout_vd_bus_1_out_31117 : Outport
  wires:
  State_vd_bus_1_cf04b/1 -> Blockout_vd_bus_1_out_31117/1

== system case1/AC_1/vd_bus_2_out_block ==
  note: vd_bus_2_out in case1
      | $\mathrm{vd}_{\mathrm{bus},2}$
      | Automatically generated on 2025-10-31 18:51:05 .
  State_vd_bus_2_8d3e6 : Inport
  Blockout_vd_bus_2_out_8740e : Outport
  wires:
  State_vd_bus_2_8d3e6/1 -> Blockout_vd_bus_2_out_8740e/1

== system case1/AC_1/vd_bus_3_out_block ==
  note: vd_bus_3_out in case1
      | $\mathrm{vd}_{\mathrm{bus},3}$
      | Automatically generated on 2025-10-31 18:51:08 .
  State_vd_bus_3_84175 : Inport
  Blockout_vd_bus_3_out_e6f06 : Outport
  wires:
  State_vd_bus_3_84175/1 -> Blockout_vd_bus_3_out_e6f06/1

== system case1/AC_1/vq_bus_1_out_block ==
  note: vq_bus_1_out in case1
      | $\mathrm{vq}_{\mathrm{bus},1}$
      | Automatically generated on 2025-10-31 18:51:03 .
  State_vq_bus_1_2880f : Inport
  Blockout_vq_bus_1_out_f8f58 : Outport
  wires:
  State_vq_bus_1_2880f/1 -> Blockout_vq_bus_1_out_f8f58/1

== system case1/AC_1/vq_bus_2_out_block ==
  note: vq_bus_2_out in case1
      | $\mathrm{vq}_{\mathrm{bus},2}$
      | Automatically generated on 2025-10-31 18:51:06 .
  State_vq_bus_2_101ce : Inport
  Blockout_vq_bus_2_out_5caa2 : Outport
  wires:
  State_vq_bus_2_101ce/1 -> Blockout_vq_bus_2_out_5caa2/1

== system case1/AC_1/vq_bus_3_out_block ==
  note: vq_bus_3_out in case1
      | $\mathrm{vq}_{\mathrm{bus},3}$
      | Automatically generated on 2025-10-31 18:51:08 .
  State_vq_bus_3_18347 : Inport
  Blockout_vq_bus_3_out_93aa3 : Outport
  wires:
  State_vq_bus_3_18347/1 -> Blockout_vq_bus_3_out_93aa3/1

== system case1/SG_D_1/T_e_SG_D_1_block ==
  note: T_e_SG_D_1 in case1
      | $-\frac{\psi _{d,\mathrm{SG},D,1}\,\left(\psi _{q,\mathrm{SG},D,1}+\frac{\psi _{\mathrm{gq},\mathrm{SG},D,1}\,\left(x_{l}-x_{\mathrm{qdd}}\right)}{x_{l}-x_{\mathrm{qd}}}+\frac{\psi _{\mathrm{kq},\mathrm{SG},D,1}\,\left(x_{\mathrm{qd}}-x_{\mathrm{qdd}}\right)}{x_{l}-x_{\mathrm{qd}}}\right)}{x_{\mathrm{qdd}}}-\frac{\psi _{q,\mathrm{SG},D,1}\,\left(\frac{\psi _{\mathrm{1d},\mathrm{SG},D,1}\,\left(x_{\mathrm{dd}}-x_{\mathrm{ddd}}\right)}{x_{\mathrm{dd}}-x_{l}}-\psi _{d,\mathrm{SG},D,1}+\frac{\psi _{\mathrm{fd},\mathrm{SG},D,1}\,\left(x_{\mathrm{ddd}}-x_{l}\right)}{x_{\mathrm{dd}}-x_{l}}\right)}{x_{\mathrm{ddd}}}$
      | Automatically generated on 2025-10-31 18:47:55 .
  State_psi_d_SG_D_1_20e40 : Inport
  State_psi_gq_SG_D_1_ab29c : Inport  Port=2
  State_psi_kq_SG_D_1_ea1db : Inport  Port=3
  State_psi_q_SG_D_1_7ae8a : Inport  Port=4
  State_psi_q_SG_D_1_09903 : Inport  Port=5
  State_psi_1d_SG_D_1_b2d45 : Inport  Port=6
  State_psi_d_SG_D_1_5ffcd : Inport  Port=7
  State_psi_fd_SG_D_1_41c9f : Inport  Port=8
  Add_1cabd : Sum
  Add_446d7 : Sum
  Add_4c533 : Sum
  Add_5b3d9 : Sum
  Add_d8b68 : Sum
  Add_ed9a0 : Sum
  Constant_-1_04413 : Constant  Value=-1
  Constant_-1_11c1e : Constant  Value=-1
  Constant_-1_16269 : Constant  Value=-1
  Constant_-1_7602b : Constant  Value=-1
  Constant_-1_a890a : Constant  Value=-1
  Constant_x_dd_d53e3 : Constant  Value=x_dd
  Constant_x_dd_f6e91 : Constant  Value=x_dd
  Constant_x_dd_feb88 : Constant  Value=x_dd
  Constant_x_ddd_3feba : Constant  Value=x_ddd
  Constant_x_ddd_a0222 : Constant  Value=x_ddd
  Constant_x_ddd_bfc7d : Constant  Value=x_ddd
  Constant_x_l_00b8a : Constant  Value=x_l
  Constant_x_l_2735a : Constant  Value=x_l
  Constant_x_l_3f8dd : Constant  Value=x_l
  Constant_x_l_40eee : Constant  Value=x_l
  Constant_x_l_b7248 : Constant  Value=x_l
  Constant_x_l_e302f : Constant  Value=x_l
  Constant_x_qd_0a56a : Constant  Value=x_qd
  Constant_x_qd_e23b5 : Constant  Value=x_qd
  Constant_x_qd_f400f : Constant  Value=x_qd
  Constant_x_qdd_3fcfd : Constant  Value=x_qdd
  Constant_x_qdd_75c6e : Constant  Value=x_qdd
  Constant_x_qdd_77ac2 : Constant  Value=x_qdd
  Divide_39fb7 : Product  Inputs=*/
  Divide_768d9 : Product  Inputs=*/
  Divide_78f8d : Product  Inputs=*/
  Divide_accd6 : Product  Inputs=*/
  Divide_dc5b3 : Product  Inputs=*/
  Divide_e6706 : Product  Inputs=*/
  Product_016f1 : Product
  Product_05314 : Product
  Product_2367e : Product
  Product_41415 : Product
  Product_75e24 : Product
  Product_83995 : Product
  Product_b4455 : Product
  Product_bd2f3 : Product
  Product_bead9 : Product
  Product_c499e : Product
  Product_ee5cb : Product
  Subtract_0f698 : Sum  Inputs=+-
  Subtract_23e18 : Sum  Inputs=+-
  Subtract_61cda : Sum  Inputs=+-
  Subtract_7d36f : Sum  Inputs=+-
  Subtract_909f1 : Sum  Inputs=+-
  Subtract_b64fd : Sum  Inputs=+-
  Subtract_bbea6 : Sum  Inputs=+-
  Blockout_T_e_SG_D_1_92784 : Outport
  wires:
  Product_41415/1 -> Divide_accd6/1
  Product_ee5cb/1 -> Add_4c533/1
  Divide_accd6/1 -> Subtract_7d36f/1
  Constant_-1_16269/1 -> Product_ee5cb/1
  Constant_x_l_e302f/1 -> Product_ee5cb/2
  Constant_x_qdd_3fcfd/1 -> Add_4c533/2
  Constant_x_qd_f400f/1 -> Subtract_61cda/1
  Constant_-1_7602b/1 -> Product_bead9/1
  Constant_x_qdd_75c6e/1 -> Divide_78f8d/2
  Constant_x_qdd_77ac2/1 -> Subtract_61cda/2
  State_psi_q_SG_D_1_09903/1 -> Product_016f1/1
  Constant_x_dd_d53e3/1 -> Subtract_bbea6/1
  Constant_x_l_b7248/1 -> Product_bead9/2
  Subtract_bbea6/1 -> Product_75e24/2
  Constant_-1_a890a/1 -> Product_b4455/1
  Constant_x_l_2735a/1 -> Product_b4455/2
  Subtract_0f698/1 -> Product_016f1/2
  State_psi_q_SG_D_1_7ae8a/1 -> Add_1cabd/2
  Constant_-1_11c1e/1 -> Product_bd2f3/1
  State_psi_1d_SG_D_1_b2d45/1 -> Product_bd2f3/2
  Constant_x_ddd_3feba/1 -> Subtract_bbea6/2
  State_psi_gq_SG_D_1_ab29c/1 -> Product_41415/1
  Add_4c533/1 -> Product_41415/2
  Product_bead9/1 -> Add_446d7/1
  Product_c499e/1 -> Product_2367e/1
  Constant_x_qd_0a56a/1 -> Add_446d7/2
  Product_75e24/1 -> Divide_39fb7/1
  State_psi_kq_SG_D_1_ea1db/1 -> Product_05314/1
  Add_446d7/1 -> Divide_accd6/2
  Subtract_61cda/1 -> Product_05314/2
  Product_b4455/1 -> Add_ed9a0/1
  Constant_x_qd_e23b5/1 -> Add_ed9a0/2
  Product_05314/1 -> Divide_768d9/1
  Product_bd2f3/1 -> Product_75e24/1
  Constant_x_dd_f6e91/1 -> Subtract_23e18/1
  Constant_x_l_3f8dd/1 -> Subtract_23e18/2
  Constant_x_ddd_a0222/1 -> Subtract_909f1/1
  Product_016f1/1 -> Divide_e6706/1
  Constant_x_l_00b8a/1 -> Subtract_909f1/2
  Divide_78f8d/1 -> Add_d8b68/1
  Product_2367e/1 -> Divide_78f8d/1
  Add_ed9a0/1 -> Divide_768d9/2
  Subtract_7d36f/1 -> Add_1cabd/1
  Divide_768d9/1 -> Subtract_7d36f/2
  Subtract_23e18/1 -> Divide_39fb7/2
  State_psi_fd_SG_D_1_41c9f/1 -> Product_83995/1
  Constant_x_ddd_bfc7d/1 -> Divide_e6706/2
  Subtract_909f1/1 -> Product_83995/2
  Constant_x_dd_feb88/1 -> Subtract_b64fd/1
  Constant_x_l_40eee/1 -> Subtract_b64fd/2
  Divide_39fb7/1 -> Add_5b3d9/1
  Add_5b3d9/1 -> Subtract_0f698/1
  State_psi_d_SG_D_1_5ffcd/1 -> Add_5b3d9/2
  Product_83995/1 -> Divide_dc5b3/1
  Subtract_b64fd/1 -> Divide_dc5b3/2
  Constant_-1_04413/1 -> Product_c499e/1
  State_psi_d_SG_D_1_20e40/1 -> Product_c499e/2
  Divide_dc5b3/1 -> Subtract_0f698/2
  Add_1cabd/1 -> Product_2367e/2
  Divide_e6706/1 -> Add_d8b68/2
  Add_d8b68/1 -> Blockout_T_e_SG_D_1_92784/1

== system case1/SG_D_1/d_E_fd_SG_D_1_block ==
  note: d_E_fd_SG_D_1 in case1
      | $\frac{V_{f,\mathrm{SG},D,1}-E_{\mathrm{fd},\mathrm{SG},D,1}\,K_{E}}{T_{E}}$
      | Automatically generated on 2025-10-31 18:47:36 .
  State_E_fd_SG_D_1_abc9a : Inport
  State_V_f_SG_D_1_13267 : Inport  Port=2
  Add_d8e39 : Sum
  Constant_-1_526da : Constant  Value=-1
  Constant_K_E_49e68 : Constant  Value=K_E
  Constant_T_E_7b94d : Constant  Value=T_E
  Divide_8b41b : Product  Inputs=*/
  Product_8721c : Product
  Product_891be : Product
  Blockout_d_E_fd_SG_D_1_97a11 : Outport
  wires:
  Add_d8e39/1 -> Divide_8b41b/1
  Constant_-1_526da/1 -> Product_891be/1
  State_E_fd_SG_D_1_abc9a/1 -> Product_891be/2
  Product_891be/1 -> Product_8721c/1
  Constant_K_E_49e68/1 -> Product_8721c/2
  Product_8721c/1 -> Add_d8e39/1
  Constant_T_E_7b94d/1 -> Divide_8b41b/2
  State_V_f_SG_D_1_13267/1 -> Add_d8e39/2
  Divide_8b41b/1 -> Blockout_d_E_fd_SG_D_1_97a11/1

== system case1/SG_D_1/d_Px_1_SG_D_1_block ==
  note: d_Px_1_SG_D_1 in case1
      | $\frac{w_{\mathrm{SG},D,1}-2\,\pi \,f_{0}}{T_{w}}-\frac{\mathrm{Px}_{1,\mathrm{SG},D,1}}{T_{w}}$
      | Automatically generated on 2025-10-31 18:47:37 .
  State_Px_1_SG_D_1_f6150 : Inport
  State_w_SG_D_1_7a36e : Inport  Port=2
  Add_214fc : Sum
  Add_67e70 : Sum
  Constant_-1_1c1b5 : Constant  Value=-1
  Constant_-2.0_83634 : Constant  Value=-2.0
  Constant_T_w_4cee7 : Constant  Value=T_w
  Constant_T_w_a8a1a : Constant  Value=T_w
  Constant_f0_58562 : Constant  Value=f0
  Constant_pi_10227 : Constant  Value=pi
  Divide_b7725 : Product  Inputs=*/
  Divide_e5f13 : Product  Inputs=*/
  Product_348ec : Product
  Product_34dc5 : Product
  Product_a91d0 : Product
  Blockout_d_Px_1_SG_D_1_e6c1c : Outport
  wires:
  Add_214fc/1 -> Blockout_d_Px_1_SG_D_1_e6c1c/1
  Constant_-2.0_83634/1 -> Product_34dc5/1
  Product_348ec/1 -> Divide_b7725/1
  State_w_SG_D_1_7a36e/1 -> Add_67e70/2
  Constant_-1_1c1b5/1 -> Product_348ec/1
  Constant_f0_58562/1 -> Product_a91d0/2
  Constant_pi_10227/1 -> Product_34dc5/2
  Product_a91d0/1 -> Add_67e70/1
  Product_34dc5/1 -> Product_a91d0/1
  State_Px_1_SG_D_1_f6150/1 -> Product_348ec/2
  Constant_T_w_a8a1a/1 -> Divide_b7725/2
  Add_67e70/1 -> Divide_e5f13/1
  Constant_T_w_4cee7/1 -> Divide_e5f13/2
  Divide_b7725/1 -> Add_214fc/1
  Divide_e5f13/1 -> Add_214fc/2

== system case1/SG_D_1/d_Px_2_SG_D_1_block ==
  note: d_Px_2_SG_D_1 in case1
      | $\frac{\mathrm{Px}_{1,\mathrm{SG},D,1}-T_{2}\,\left(\frac{\mathrm{Px}_{1,\mathrm{SG},D,1}}{T_{w}}-\frac{w_{\mathrm{SG},D,1}-2\,\pi \,f_{0}}{T_{w}}\right)}{T_{1}}-\frac{\mathrm{Px}_{2,\mathrm{SG},D,1}}{T_{1}}$
      | Automatically generated on 2025-10-31 18:47:39 .
  State_Px_2_SG_D_1_48e57 : Inport
  State_Px_1_SG_D_1_f11fa : Inport  Port=2
  State_Px_1_SG_D_1_b3d15 : Inport  Port=3
  State_w_SG_D_1_5d530 : Inport  Port=4
  Add_1dd20 : Sum
  Add_eab54 : Sum
  Add_f7360 : Sum
  Add_fe257 : Sum
  Constant_-1_0f729 : Constant  Value=-1
  Constant_-1_ddc81 : Constant  Value=-1
  Constant_-2.0_a7dc9 : Constant  Value=-2.0
  Constant_T_1_5b5ce : Constant  Value=T_1
  Constant_T_1_ea562 : Constant  Value=T_1
  Constant_T_2_2f774 : Constant  Value=T_2
  Constant_T_w_7aff8 : Constant  Value=T_w
  Constant_T_w_fba6d : Constant  Value=T_w
  Constant_f0_dbabd : Constant  Value=f0
  Constant_pi_9a422 : Constant  Value=pi
  Divide_09798 : Product  Inputs=*/
  Divide_a7d64 : Product  Inputs=*/
  Divide_e342a : Product  Inputs=*/
  Divide_ed738 : Product  Inputs=*/
  Product_11522 : Product
  Product_3c33f : Product
  Product_8a59b : Product
  Product_d3713 : Product
  Product_fd057 : Product
  Blockout_d_Px_2_SG_D_1_4e1cd : Outport
  wires:
  Constant_-2.0_a7dc9/1 -> Product_8a59b/1
  State_w_SG_D_1_5d530/1 -> Add_f7360/2
  Constant_f0_dbabd/1 -> Product_11522/2
  Constant_pi_9a422/1 -> Product_8a59b/2
  Add_1dd20/1 -> Product_d3713/2
  Product_11522/1 -> Add_f7360/1
  Divide_e342a/1 -> Add_1dd20/1
  Product_8a59b/1 -> Product_11522/1
  Constant_T_w_7aff8/1 -> Divide_e342a/2
  Constant_-1_0f729/1 -> Product_fd057/1
  State_Px_1_SG_D_1_b3d15/1 -> Product_fd057/2
  Divide_ed738/1 -> Add_fe257/1
  Product_fd057/1 -> Divide_e342a/1
  Add_f7360/1 -> Divide_a7d64/1
  Constant_T_w_fba6d/1 -> Divide_a7d64/2
  Divide_a7d64/1 -> Add_1dd20/2
  Constant_T_2_2f774/1 -> Product_d3713/1
  Constant_-1_ddc81/1 -> Product_3c33f/1
  State_Px_2_SG_D_1_48e57/1 -> Product_3c33f/2
  State_Px_1_SG_D_1_f11fa/1 -> Add_eab54/1
  Product_d3713/1 -> Add_eab54/2
  Add_eab54/1 -> Divide_09798/1
  Product_3c33f/1 -> Divide_ed738/1
  Constant_T_1_ea562/1 -> Divide_ed738/2
  Constant_T_1_5b5ce/1 -> Divide_09798/2
  Divide_09798/1 -> Add_fe257/2
  Add_fe257/1 -> Blockout_d_Px_2_SG_D_1_4e1cd/1

== system case1/SG_D_1/d_Px_3_SG_D_1_block ==
  note: d_Px_3_SG_D_1 in case1
      | $\frac{\mathrm{Px}_{2,\mathrm{SG},D,1}+T_{4}\,\left(\frac{\mathrm{Px}_{1,\mathrm{SG},D,1}-T_{2}\,\left(\frac{\mathrm{Px}_{1,\mathrm{SG},D,1}}{T_{w}}-\frac{w_{\mathrm{SG},D,1}-2\,\pi \,f_{0}}{T_{w}}\right)}{T_{1}}-\frac{\mathrm{Px}_{2,\mathrm{SG},D,1}}{T_{1}}\right)}{T_{3}}-\frac{\mathrm{Px}_{3,\mathrm{SG},D,1}}{T_{3}}$
      | Automatically generated on 2025-10-31 18:47:42 .
  State_Px_3_SG_D_1_4be19 : Inport
  State_Px_2_SG_D_1_f2fa6 : Inport  Port=2
  State_Px_2_SG_D_1_adf7b : Inport  Port=3
  State_Px_1_SG_D_1_e02b1 : Inport  Port=4
  State_Px_1_SG_D_1_a6ed2 : Inport  Port=5
  State_w_SG_D_1_55a2f : Inport  Port=6
  Add_19047 : Sum
  Add_35bdc : Sum
  Add_875ad : Sum
  Add_8b05e : Sum
  Add_9784b : Sum
  Add_e275b : Sum
  Constant_-1_26313 : Constant  Value=-1
  Constant_-1_2ba91 : Constant  Value=-1
  Constant_-1_5e1fd : Constant  Value=-1
  Constant_-2.0_3ec9e : Constant  Value=-2.0
  Constant_T_1_0c170 : Constant  Value=T_1
  Constant_T_1_3bca1 : Constant  Value=T_1
  Constant_T_2_ab1bc : Constant  Value=T_2
  Constant_T_3_281a6 : Constant  Value=T_3
  Constant_T_3_c1628 : Constant  Value=T_3
  Constant_T_4_f41ce : Constant  Value=T_4
  Constant_T_w_39805 : Constant  Value=T_w
  Constant_T_w_e659c : Constant  Value=T_w
  Constant_f0_55085 : Constant  Value=f0
  Constant_pi_c8dd1 : Constant  Value=pi
  Divide_0d389 : Product  Inputs=*/
  Divide_29d9f : Product  Inputs=*/
  Divide_3cf14 : Product  Inputs=*/
  Divide_51d8d : Product  Inputs=*/
  Divide_65128 : Product  Inputs=*/
  Divide_c9961 : Product  Inputs=*/
  Product_1535d : Product
  Product_25017 : Product
  Product_508f3 : Product
  Product_7d673 : Product
  Product_870b2 : Product
  Product_87e9b : Product
  Product_9456d : Product
  Blockout_d_Px_3_SG_D_1_8cb1d : Outport
  wires:
  Constant_T_w_39805/1 -> Divide_c9961/2
  Constant_-1_26313/1 -> Product_87e9b/1
  Add_35bdc/1 -> Blockout_d_Px_3_SG_D_1_8cb1d/1
  Constant_-2.0_3ec9e/1 -> Product_1535d/1
  State_w_SG_D_1_55a2f/1 -> Add_9784b/2
  Constant_f0_55085/1 -> Product_870b2/2
  State_Px_1_SG_D_1_a6ed2/1 -> Product_87e9b/2
  Constant_pi_c8dd1/1 -> Product_1535d/2
  Product_870b2/1 -> Add_9784b/1
  Product_1535d/1 -> Product_870b2/1
  Product_87e9b/1 -> Divide_c9961/1
  Divide_51d8d/1 -> Add_35bdc/1
  Constant_T_3_c1628/1 -> Divide_0d389/2
  Add_9784b/1 -> Divide_29d9f/1
  Constant_T_w_e659c/1 -> Divide_29d9f/2
  Divide_c9961/1 -> Add_8b05e/1
  Divide_29d9f/1 -> Add_8b05e/2
  Constant_-1_5e1fd/1 -> Product_25017/1
  Constant_T_2_ab1bc/1 -> Product_7d673/1
  Add_8b05e/1 -> Product_7d673/2
  Constant_-1_2ba91/1 -> Product_9456d/1
  Divide_0d389/1 -> Add_35bdc/2
  Constant_T_3_281a6/1 -> Divide_51d8d/2
  State_Px_2_SG_D_1_adf7b/1 -> Product_9456d/2
  State_Px_1_SG_D_1_e02b1/1 -> Add_e275b/1
  Divide_65128/1 -> Add_875ad/1
  Product_7d673/1 -> Add_e275b/2
  Product_9456d/1 -> Divide_65128/1
  Product_25017/1 -> Divide_51d8d/1
  Constant_T_1_3bca1/1 -> Divide_65128/2
  Add_e275b/1 -> Divide_3cf14/1
  Constant_T_1_0c170/1 -> Divide_3cf14/2
  Divide_3cf14/1 -> Add_875ad/2
  Constant_T_4_f41ce/1 -> Product_508f3/1
  Add_875ad/1 -> Product_508f3/2
  State_Px_3_SG_D_1_4be19/1 -> Product_25017/2
  State_Px_2_SG_D_1_f2fa6/1 -> Add_19047/1
  Product_508f3/1 -> Add_19047/2
  Add_19047/1 -> Divide_0d389/1

== system case1/SG_D_1/d_R_f_SG_D_1_block ==
  note: d_R_f_SG_D_1 in case1
      | $-\frac{R_{f,\mathrm{SG},D,1}-\frac{E_{\mathrm{fd},\mathrm{SG},D,1}\,K_{F}}{T_{F}}}{T_{F}}$
      | Automatically generated on 2025-10-31 18:47:35 .
  State_E_fd_SG_D_1_eb437 : Inport
  State_R_f_SG_D_1_00ad4 : Inport  Port=2
  Constant_K_F_f556c : Constant  Value=K_F
  Constant_T_F_152a2 : Constant  Value=T_F
  Constant_T_F_42b04 : Constant  Value=T_F
  Divide_1faee : Product  Inputs=*/
  Divide_d8e3d : Product  Inputs=*/
  Product_2320b : Product
  Subtract_06fe2 : Sum  Inputs=+-
  Blockout_d_R_f_SG_D_1_76ad3 : Outport
  wires:
  Constant_K_F_f556c/1 -> Product_2320b/2
  Product_2320b/1 -> Divide_d8e3d/1
  State_E_fd_SG_D_1_eb437/1 -> Product_2320b/1
  State_R_f_SG_D_1_00ad4/1 -> Subtract_06fe2/2
  Constant_T_F_42b04/1 -> Divide_d8e3d/2
  Divide_d8e3d/1 -> Subtract_06fe2/1
  Divide_1faee/1 -> Blockout_d_R_f_SG_D_1_76ad3/1
  Subtract_06fe2/1 -> Divide_1faee/1
  Constant_T_F_152a2/1 -> Divide_1faee/2

== system case1/SG_D_1/d_T_m_SG_D_1_block ==
  note: d_T_m_SG_D_1 in case1
      | $-\frac{T_{m,\mathrm{SG},D,1}-T_{0}+\frac{\mathrm{SpeedPara}\,\left(w_{\mathrm{SG},D,1}-w_{\mathrm{ref}}\right)}{2\,f_{0}\,\pi }}{T_{\mathrm{speed}}}$
      | Automatically generated on 2025-10-31 18:47:25 .
  State_w_SG_D_1_c2877 : Inport
  State_T_m_SG_D_1_3f3eb : Inport  Port=2
  Add_72198 : Sum
  Add_837cc : Sum
  Constant_-1_f5a6d : Constant  Value=-1
  Constant_2.0_d2fb2 : Constant  Value=2.0
  Constant_SpeedPara_e9f3b : Constant  Value=SpeedPara
  Constant_T_0_b423d : Constant  Value=T_0
  Constant_T_speed_483f0 : Constant  Value=T_speed
  Constant_f0_14912 : Constant  Value=f0
  Constant_pi_0b8b8 : Constant  Value=pi
  Constant_w_ref_df6f6 : Constant  Value=w_ref
  Divide_0694e : Product  Inputs=*/
  Divide_a94c0 : Product  Inputs=*/
  Product_7d47e : Product
  Product_b7659 : Product
  Product_b8d92 : Product
  Product_d4ff1 : Product
  Subtract_439ad : Sum  Inputs=+-
  Blockout_d_T_m_SG_D_1_7bd94 : Outport
  wires:
  Constant_-1_f5a6d/1 -> Product_b8d92/1
  Constant_w_ref_df6f6/1 -> Add_72198/2
  State_w_SG_D_1_c2877/1 -> Product_b8d92/2
  Add_837cc/1 -> Subtract_439ad/1
  Add_72198/1 -> Product_7d47e/2
  Product_b8d92/1 -> Add_72198/1
  Constant_2.0_d2fb2/1 -> Product_b7659/1
  Constant_pi_0b8b8/1 -> Product_b7659/2
  Constant_SpeedPara_e9f3b/1 -> Product_7d47e/1
  Product_b7659/1 -> Product_d4ff1/1
  Constant_f0_14912/1 -> Product_d4ff1/2
  Constant_T_speed_483f0/1 -> Divide_0694e/2
  Product_7d47e/1 -> Divide_a94c0/1
  Product_d4ff1/1 -> Divide_a94c0/2
  Divide_a94c0/1 -> Add_837cc/1
  Constant_T_0_b423d/1 -> Add_837cc/2
  State_T_m_SG_D_1_3f3eb/1 -> Subtract_439ad/2
  Subtract_439ad/1 -> Divide_0694e/1
  Divide_0694e/1 -> Blockout_d_T_m_SG_D_1_7bd94/1
